simulink subsystem "Rain"  (R2025b)
settings: Solver=VariableStepAuto  StartTime=0.0  StopTime=10.0  RelTol=1e-3
model mask{Duration=10, Flowrate=1, BurstStart=1, BurstFlow=1, BurstDur=1, flip_order=off, rain_start=0, station_order=0, EnableBurst=on}
  mask prompts: Flowrate "Flowrate (liters/min)"; BurstStart "Burst start:"; BurstFlow "Burst flow:"; BurstDur "Burst duration:"; flip_order "Flip order"; rain_start "Rain start (sec):"; station_order "Station order:"; EnableBurst "Enable cloud burst"
settings Model: Creator=klump  LastModifiedBy=klump

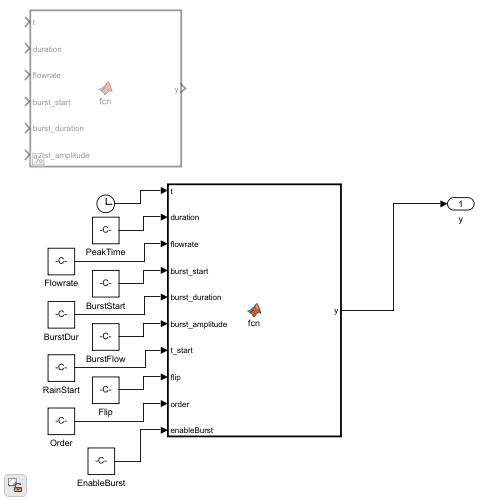
[thumbnail: Simulink's stored preview of the top-level diagram]
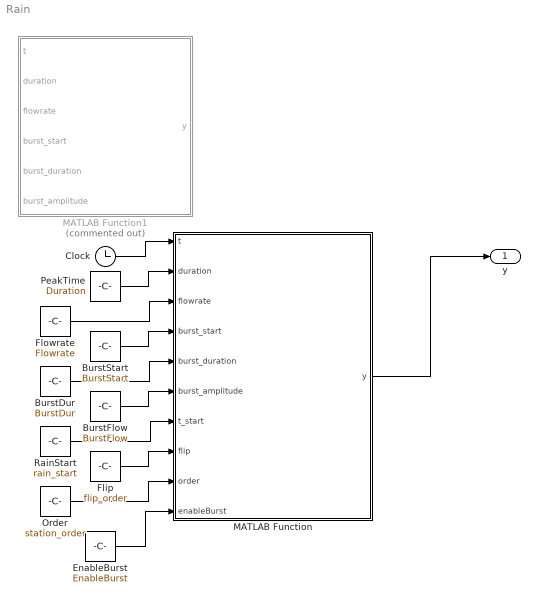
== system Rain ==
  BurstDur : Constant  Value=BurstDur
  BurstFlow : Constant  Value=BurstFlow
  BurstStart : Constant  Value=BurstStart
  Clock : Clock
  EnableBurst : Constant  Value=EnableBurst
  Flip : Constant  Value=flip_order
  Flowrate : Constant  Value=Flowrate
  MATLAB Function : MATLAB Function  TreatAsAtomicUnit=on
  MATLAB Function1 : MATLAB Function  Commented=on  TreatAsAtomicUnit=on
  Order : Constant  Value=station_order
  PeakTime : Constant  Value=Duration
  RainStart : Constant  Value=rain_start
  y : Outport
  wires:
  EnableBurst/1 -> MATLAB Function/10(enableBurst)
  Order/1 -> MATLAB Function/9(order)
  Flip/1 -> MATLAB Function/8(flip)
  RainStart/1 -> MATLAB Function/7(t_start)
  PeakTime/1 -> MATLAB Function/2(duration)
  Clock/1 -> MATLAB Function/1(t)
  MATLAB Function/1(y) -> y/1
  Flowrate/1 -> MATLAB Function/3(flowrate)
  BurstFlow/1 -> MATLAB Function/6(burst_amplitude)
  BurstStart/1 -> MATLAB Function/4(burst_start)
  BurstDur/1 -> MATLAB Function/5(burst_duration)

== matlab function Rain/MATLAB Function ==
  data: t input; y output; duration input; flowrate input; burst_start input; burst_duration input; burst_amplitude input; t_start input; flip input; order input; enableBurst input
function y = fcn(t,duration, flowrate, burst_start,burst_duration, burst_amplitude,t_start, flip, order,enableBurst)
%flowrate
    if flip
        order = 5-order;
    end
    t_start= t_start*order;
    %burst_start = burst_start + t_start;
    burst_start = t_start + duration/2 - burst_duration/2; %0.5*burst_start*order;%+t_start;

    
    if (duration+t_start > t) && (t >= t_start) && (((burst_start > t) || (burst_duration+burst_start <= t)) || (burst_amplitude < flowrate) ||  ~enableBurst )
        y = flowrate/60;     
    elseif (burst_start >= t_start) && (burst_start <= t) && (burst_duration+burst_start > t) && (burst_amplitude > flowrate) && enableBurst
        y = burst_amplitude/60;    
    else
        y = 0;
    end
        

    
end

== matlab function Rain/MATLAB Function1 ==
  data: t input; y output; duration input; flowrate input; burst_start input; burst_duration input; burst_amplitude input
function y = fcn(t,duration, flowrate, burst_start,burst_duration, burst_amplitude)
%flowrate
if (duration > t) && (t >= 0)
    %disp("rain")
    %y = 1/(duration * flowrate/60*((24.5/2)*10)^2*pi*0.000001);
    if (burst_start < t) && (burst_duration+burst_start > t) && (burst_amplitude > flowrate)
        y = burst_amplitude/60;
    else
        y = flowrate/60;
    end
else
    %disp("No rain")

    y = 0;
end
